simulink model "test"  (R2023b)
settings: Solver=VariableStepAuto  StartTime=0.0  StopTime=10.0  RelTol=1e-3
settings Model: Creator=admin  LastModifiedBy=admin

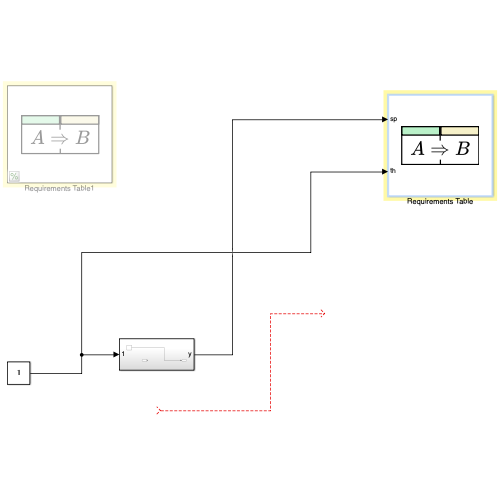
[thumbnail: Simulink's stored preview of the top-level diagram]
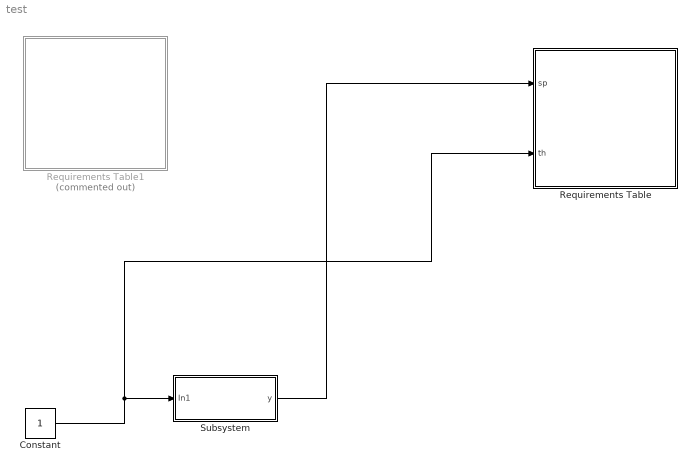
== system test ==
  Constant : Constant
  Requirements Table : Requirements Table  TreatAsAtomicUnit=on
  Requirements Table1 : Requirements Table  Commented=on  TreatAsAtomicUnit=on
  Subsystem : Subsystem
  wires:
  Constant/1 -> Subsystem/1(In1), Requirements Table/2(th)
  ? -> ?
  Subsystem/1(y) -> Requirements Table/1(sp)

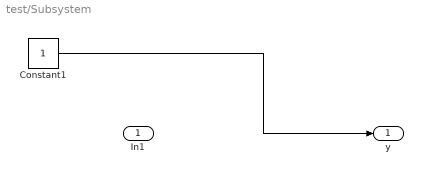
== system test/Subsystem ==
  In1 : Inport
  Constant1 : Constant
  y : Outport
  wires:
  Constant1/1 -> y/1

== stateflow chart test/Requirements Table1 ==
  (default) -> (junction 1073741860)
  (junction 1073741860) -> (junction 1073741861) : {
      | % SF_REQ_REV_07
      | }
  (junction 1073741861) -> (junction 1073741863) : {
      | % HEADER_ASSIGNMENTS
      |
      | }
  (junction 1073741863) -> (junction 1073741865) : {
      | % START_A_4
      | }
  (junction 1073741865) -> (junction 1073741867) : {
      | }
  (junction 1073741867) -> (junction 1073741869)
  (junction 1073741869) -> (junction 1073741871) : {
      | }
  (junction 1073741871) -> (junction 1073741873) : {
      | % END_A_4
      | }
  (junction 1073741873) -> (junction 1073741898) : {
      | % START_R_1
      | }
  (junction 1073741898) -> (junction 1073741900) : {
      | }
  (junction 1073741900) -> (junction 1073741902) : {
      |
      |
      | }
  (junction 1073741902) -> (junction 1073741904) : {
      | }
  (junction 1073741904) -> (junction 1073741906) : {
      | % END_R_1
      | }

== stateflow chart test/Requirements Table ==
  (default) -> (junction 1073741860)
  (junction 1073741860) -> (junction 1073741861) : {
      | % SF_REQ_REV_07
      | }
  (junction 1073741861) -> (junction 1073741863) : {
      | % HEADER_ASSIGNMENTS
      |
      | }
  (junction 1073741863) -> (junction 1073741865) : {
      | % START_A_4
      | }
  (junction 1073741865) -> (junction 1073741867) : {
      | }
  (junction 1073741867) -> (junction 1073741869)
  (junction 1073741869) -> (junction 1073741871) : {
      | }
  (junction 1073741871) -> (junction 1073741873) : {
      | % END_A_4
      | }
  (junction 1073741873) -> (junction 1073741925) : {
      | % START_R_1
      | }
  (junction 1073741925) -> (junction 1073741927) : {
      | }
  (junction 1073741927) -> (junction 1073741929)
  (junction 1073741929) -> (junction 1073741931) [order 1] : [(th>0)]
  (junction 1073741929) -> (junction 1073741937) [order 2]
  (junction 1073741931) -> (junction 1073741933) : {
      | reqtable_postcondition((sp==prev(sp)+th), 'R:1');
      |
      |
      | }
  (junction 1073741933) -> (junction 1073741935) : {
      | }
  (junction 1073741935) -> (junction 1073741937)
  (junction 1073741937) -> (junction 1073741939)
  (junction 1073741939) -> (junction 1073741941) : {
      | % END_R_1
      | }
  (junction 1073741941) -> (junction 1073741950) : {
      | % START_R_7
      | }
  (junction 1073741950) -> (junction 1073741952) : {
      | }
  (junction 1073741952) -> (junction 1073741954)
  (junction 1073741954) -> (junction 1073741956) [order 1] : [(prev(sp)==160)]
  (junction 1073741954) -> (junction 1073741962) [order 2]
  (junction 1073741956) -> (junction 1073741958) : {
      | reqtable_postcondition((sp<10), 'R:2');
      |
      |
      | }
  (junction 1073741958) -> (junction 1073741960) : {
      | }
  (junction 1073741960) -> (junction 1073741962)
  (junction 1073741962) -> (junction 1073741964)
  (junction 1073741964) -> (junction 1073741966) : {
      | % END_R_7
      | }
  (junction 1073741966) -> (junction 1073741983) : {
      | % START_R_10
      | }
  (junction 1073741983) -> (junction 1073741985) : {
      | }
  (junction 1073741985) -> (junction 1073741987)
  (junction 1073741987) -> (junction 1073741989) [order 1] : [(th<0)]
  (junction 1073741987) -> (junction 1073741995) [order 2]
  (junction 1073741989) -> (junction 1073741991) : {
      | reqtable_postcondition((sp<prev(sp)), 'R:3');
      |
      |
      | }
  (junction 1073741991) -> (junction 1073741993) : {
      | }
  (junction 1073741993) -> (junction 1073741995)
  (junction 1073741995) -> (junction 1073741997)
  (junction 1073741997) -> (junction 1073741999) : {
      | % END_R_10
      | }
  data: sp input; th input
